simulink model "main"  (R2021a)
settings: Solver=ode113  StartTime=0.0  StopTime=100  RelTol=1e-13  AbsTol=1e-14
undefined symbols (not defined in the file or in its folder): Earth, initCond, Sensors, Spacecraft
libraries: aerolibutil x48, vrlib x31, dspsrcs4 x29, simulink x10, SADlibrary x8, commfilt2 x3, sharedtransform x3, dspfdesign x3, sharedutil x2, sharedTrackingLibrary x2, dspmathops x1
(part 2 of 3)

== system main/Subsystem1/Sun sensor reading3 ==
  True Sun position [body reference frame][km] : Inport  OutDataTypeStr=double  Unit=km
  q_S/B : Inport  Port=2
  Atan3 : Trigonometry  Operator=atan2
  Atan4 : Trigonometry  Operator=atan2
  Demux2 : Demux  Outputs=3
  Mux1 : Mux  Inputs=2
  Normalize Vector : vrlib/Utilities/Normalize Vector  maxzero=0
  Quaternion Rotation : aerolibutil/Quaternion Rotation
  Saturation1 : Saturate  UpperLimit=Sensors.sunSensor.fow  LowerLimit=-Sensors.sunSensor.fow
  Subsystem : Subsystem
  Zero-Order Hold : ZeroOrderHold  SampleTime=1/Sensors.sunSensor.freq
  Sun angles position [sensor axis] : Outport  OutDataTypeStr=double  Unit=1
  wires:
  True Sun position [body reference frame][km]/1 -> Zero-Order Hold/1
  q_S/B/1 -> Quaternion Rotation/1
  Zero-Order Hold/1 -> Normalize Vector/1
  Normalize Vector/1 -> Quaternion Rotation/2
  Quaternion Rotation/1 -> Subsystem/1(vec)
  Demux2/3 -> Atan3/2, Atan4/2
  Demux2/1 -> Atan4/1
  Atan4/1 -> Mux1/1
  Atan3/1 -> Mux1/2
  Mux1/1 -> Saturation1/1
  Subsystem/1(vec_rot) -> Demux2/1
  Demux2/2 -> Atan3/1
  Saturation1/1 -> Sun angles position [sensor axis]/1

== system main/Subsystem1/Sun sensor reading4 ==
  True Sun position [body reference frame][km] : Inport  OutDataTypeStr=double  Unit=km
  q_S/B : Inport  Port=2
  Atan3 : Trigonometry  Operator=atan2
  Atan4 : Trigonometry  Operator=atan2
  Demux2 : Demux  Outputs=3
  Mux1 : Mux  Inputs=2
  Normalize Vector : vrlib/Utilities/Normalize Vector  maxzero=0
  Quaternion Rotation : aerolibutil/Quaternion Rotation
  Saturation1 : Saturate  UpperLimit=Sensors.sunSensor.fow  LowerLimit=-Sensors.sunSensor.fow
  Subsystem : Subsystem
  Zero-Order Hold : ZeroOrderHold  SampleTime=1/Sensors.sunSensor.freq
  Sun angles position [sensor axis] : Outport  OutDataTypeStr=double  Unit=1
  wires:
  True Sun position [body reference frame][km]/1 -> Zero-Order Hold/1
  q_S/B/1 -> Quaternion Rotation/1
  Zero-Order Hold/1 -> Normalize Vector/1
  Normalize Vector/1 -> Quaternion Rotation/2
  Quaternion Rotation/1 -> Subsystem/1(vec)
  Demux2/3 -> Atan3/2, Atan4/2
  Demux2/1 -> Atan4/1
  Atan4/1 -> Mux1/1
  Atan3/1 -> Mux1/2
  Mux1/1 -> Saturation1/1
  Subsystem/1(vec_rot) -> Demux2/1
  Demux2/2 -> Atan3/1
  Saturation1/1 -> Sun angles position [sensor axis]/1

== system main/Subsystem1/Sun sensor reading5 ==
  True Sun position [body reference frame][km] : Inport  OutDataTypeStr=double  Unit=km
  q_S/B : Inport  Port=2
  Atan3 : Trigonometry  Operator=atan2
  Atan4 : Trigonometry  Operator=atan2
  Demux2 : Demux  Outputs=3
  Mux1 : Mux  Inputs=2
  Normalize Vector : vrlib/Utilities/Normalize Vector  maxzero=0
  Quaternion Rotation : aerolibutil/Quaternion Rotation
  Saturation1 : Saturate  UpperLimit=Sensors.sunSensor.fow  LowerLimit=-Sensors.sunSensor.fow
  Subsystem : Subsystem
  Zero-Order Hold : ZeroOrderHold  SampleTime=1/Sensors.sunSensor.freq
  Sun angles position [sensor axis] : Outport  OutDataTypeStr=double  Unit=1
  wires:
  True Sun position [body reference frame][km]/1 -> Zero-Order Hold/1
  q_S/B/1 -> Quaternion Rotation/1
  Zero-Order Hold/1 -> Normalize Vector/1
  Normalize Vector/1 -> Quaternion Rotation/2
  Quaternion Rotation/1 -> Subsystem/1(vec)
  Demux2/3 -> Atan3/2, Atan4/2
  Demux2/1 -> Atan4/1
  Atan4/1 -> Mux1/1
  Atan3/1 -> Mux1/2
  Mux1/1 -> Saturation1/1
  Subsystem/1(vec_rot) -> Demux2/1
  Demux2/2 -> Atan3/1
  Saturation1/1 -> Sun angles position [sensor axis]/1

== system main/Real physics/Air drag/Air density ==
  note: Because the density is a continuous function it doesn't matter if with an Height equal to a breakpoint value (e.g. =700km) we consider a base height of 700km or a base height of 600km
  Height : Inport
  1-D Lookup Base height : Lookup_n-D  NumberOfTableDimensions=1  BreakpointsForDimension1=Earth.atm_referenceHeight  IndexSearchMethod=Evenly spaced points  BeginIndexSearchUsingPreviousIndexResult=on  Table=Earth.atm_referenceHeight  InterpMethod=Flat  ExtrapMethod=Clip  UseLastTableValue=on  InternalRulePriority=Speed  RndMeth=Simplest  InputSameDT=on
  1-D Lookup Nominal density : Lookup_n-D  NumberOfTableDimensions=1  BreakpointsForDimension1=Earth.atm_referenceHeight  IndexSearchMethod=Evenly spaced points  BeginIndexSearchUsingPreviousIndexResult=on  Table=Earth.atm_nominalDensity  InterpMethod=Flat  InternalRulePriority=Speed  RndMeth=Simplest  InputSameDT=on
  1-D Lookup Scale height : Lookup_n-D  NumberOfTableDimensions=1  BreakpointsForDimension1=Earth.atm_referenceHeight  IndexSearchMethod=Evenly spaced points  BeginIndexSearchUsingPreviousIndexResult=on  Table=Earth.atm_scaleHeight  InterpMethod=Flat  InternalRulePriority=Speed  RndMeth=Simplest  InputSameDT=on
  Divide : Product  Inputs=*/
  Exp : Math  SaturateOnIntegerOverflow=on
  Product : Product
  Sum : Sum  Inputs=-+|
  Air density : Outport
  wires:
  Height/1 -> 1-D Lookup Nominal density/1, 1-D Lookup Scale height/1, 1-D Lookup Base height/1, Sum/1
  1-D Lookup Nominal density/1 -> Product/2
  1-D Lookup Base height/1 -> Sum/2
  Sum/1 -> Divide/1
  1-D Lookup Scale height/1 -> Divide/2
  Divide/1 -> Exp/1
  Product/1 -> Air density/1
  Exp/1 -> Product/1

== system main/Real physics/Magnetic dipole/Subsystem2 ==
  q_A/B : Inport
  r_NF : Inport  Port=2
  Clock : Clock
  Gain : Gain  Gain=2*pi/Earth.siderealDay
  MATLAB Function : MATLAB Function  TreatAsAtomicUnit=on
  MATLAB Function1 : MATLAB Function  TreatAsAtomicUnit=on
  Mux : Mux  Inputs=3
  Quaternion Conjugate : aerolibutil/Quaternion Conjugate
      settings: SourceProductBaseCode=AE
  Quaternion Rotation : aerolibutil/Quaternion Rotation
  Subsystem : Subsystem
  Subsystem1 : Subsystem
  B [BF] : Outport
  wires:
  q_A/B/1 -> Subsystem/1(q_A/B)
  Clock/1 -> Gain/1
  MATLAB Function/1(Bth) -> Mux/1
  Quaternion Conjugate/1 -> Subsystem/2(q_B/C)
  r_NF/1 -> MATLAB Function1/1(r_NF)
  Gain/1 -> MATLAB Function/1(RAGreenwich)
  MATLAB Function/2(Bph) -> Mux/2
  MATLAB Function1/1(RA) -> MATLAB Function/2(RA), Subsystem1/1(RA)
  Mux/1 -> Quaternion Rotation/2
  MATLAB Function1/2(dec) -> MATLAB Function/3(dec), Subsystem1/2(dec)
  MATLAB Function1/3(r) -> MATLAB Function/4(r)
  Subsystem1/1(q_T/N) -> Quaternion Conjugate/1
  Quaternion Rotation/1 -> B [BF]/1
  Subsystem/1(q_A/C) -> Quaternion Rotation/1  "Attitude error"
  MATLAB Function/3(Br) -> Mux/3

== system main/Real physics/Rotational dynamic/Euler equations (rigid body)  ==
  note: $\dot\mathbf{\Gamma} = \left[ (-I_z+I_y) \omega_y \omega_z \quad (-I_x+I_z) \omega_z \omega_x \quad \right (-I_y+I_x) \omega_x \omega_y]^T$
      |
      | Please note that
      | $\left[b \quad c \quad a \right] = \text{Cycle_3_vector}\left([a \quad b \quad c]\right)$
  omega [body reference frame] : Inport
  External torque [body reference frame] : Inport  Port=2  Unit=N*m
  Constant : Constant  Value=Spacecraft.str.inertia
  Cycle vector{,1..3} (4 alike) : SADlibrary/Cycle vector  SystemSampleTime=-1  VariantActivationTime=update diagram  Latency=0  AutoFrameSizeCalculation=off
  Divide : Product  Inputs=*/
  Product : Product  Inputs=3
  Sum : Sum  Inputs=++|
  Sum1 : Sum  Inputs=|-+
  omega dot [body reference frame] : Outport
  wires:
  Constant/1 -> Cycle vector2/1, Divide/2
  External torque [body reference frame]/1 -> Sum/1
  Sum/1 -> Divide/1
  Divide/1 -> omega dot [body reference frame]/1
  omega [body reference frame]/1 -> Cycle vector/1
  Cycle vector2/1 -> Cycle vector3/1, Sum1/1
  Cycle vector3/1 -> Sum1/2
  Cycle vector/1 -> Cycle vector1/1, Product/2
  Cycle vector1/1 -> Product/1
  Sum1/1 -> Product/3
  Product/1 -> Sum/2

== system main/Real physics/Rotational dynamic/Kinematics with quaternions ==
  q_I/N : Inport  Unit=1
  omega [IF] : Inport  Port=2  Unit=rad/s
  Gain1 : Gain  Gain=1/2
  MATLAB Function1 : MATLAB Function  TreatAsAtomicUnit=on
  Matrix Multiply : Product  Multiplication=Matrix(*)
  q_I/N_dot : Outport
  wires:
  omega [IF]/1 -> MATLAB Function1/1(omega)
  Gain1/1 -> Matrix Multiply/1
  Matrix Multiply/1 -> q_I/N_dot/1
  MATLAB Function1/1(Omega) -> Gain1/1
  q_I/N/1 -> Matrix Multiply/2

== system main/Real physics/Rotational dynamic/getGamma0 ==
  Constant1 : Constant  Value=Spacecraft.initialKepElm.a  VectorParams1D=off
  Constant3 : Constant  Value=Spacecraft.initialKepElm.e
  Constant4 : Constant  Value=Spacecraft.initialKepElm.i
  Constant5 : Constant  Value=Spacecraft.initialKepElm.Omega
  Constant6 : Constant  Value=Spacecraft.initialKepElm.f
  Constant8 : Constant  Value=Spacecraft.initialKepElm.omega
  MATLAB Function3 : MATLAB Function  TreatAsAtomicUnit=on
  MATLAB Function4 : MATLAB Function  TreatAsAtomicUnit=on
  Terminator : Terminator
  Gamma0 : Outport
  wires:
  Constant5/1 -> MATLAB Function3/4(Omega)
  MATLAB Function4/1(Gamma0) -> Gamma0/1
  Constant6/1 -> MATLAB Function3/6(f)
  Constant8/1 -> MATLAB Function3/5(omega)
  MATLAB Function3/1(r) -> Terminator/1
  Constant1/1 -> MATLAB Function3/1(a)
  MATLAB Function3/2(v) -> MATLAB Function4/1(vG0)
  Constant4/1 -> MATLAB Function3/3(i)
  Constant3/1 -> MATLAB Function3/2(e)

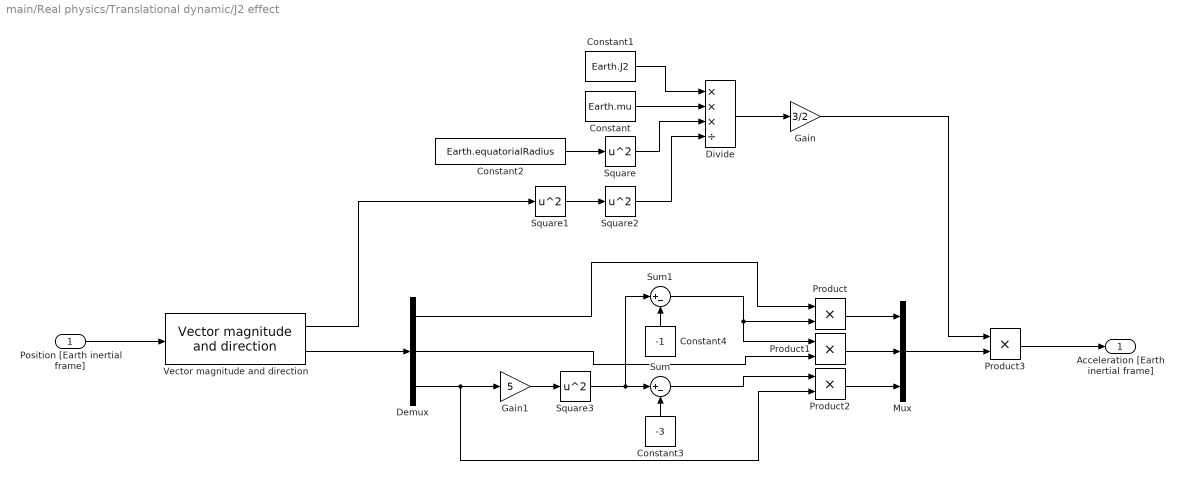
== system main/Real physics/Translational dynamic/J2 effect ==
  Position [Earth inertial frame] : Inport
  Constant : Constant  Value=Earth.mu
  Constant1 : Constant  Value=Earth.J2
  Constant2 : Constant  Value=Earth.equatorialRadius
  Constant3 : Constant  Value=-3
  Constant4 : Constant  Value=-1
  Demux : Demux  Outputs=3
  Divide : Product  Inputs=***/
  Gain : Gain  Gain=3/2
  Gain1 : Gain  Gain=5
  Mux : Mux  Inputs=3
  Product{,1..3} (4 alike) : Product
  Square{,1..3} (4 alike) : Math  Operator=square  SaturateOnIntegerOverflow=on
  Sum : Sum  Inputs=|+-
  Sum1 : Sum  Inputs=|+-
  Vector magnitude and direction : SADlibrary/Vector magnitude and direction  SystemSampleTime=-1  VariantActivationTime=update diagram  Latency=0  AutoFrameSizeCalculation=off
  Acceleration [Earth inertial frame] : Outport
  wires:
  Constant2/1 -> Square/1
  Constant1/1 -> Divide/1
  Constant/1 -> Divide/2
  Square/1 -> Divide/3
  Divide/1 -> Gain/1
  Square1/1 -> Square2/1
  Square2/1 -> Divide/4
  Vector magnitude and direction/1 -> Square1/1
  Position [Earth inertial frame]/1 -> Vector magnitude and direction/1
  Vector magnitude and direction/2 -> Demux/1
  Demux/3 -> Product2/2, Gain1/1
  Gain1/1 -> Square3/1
  Square3/1 -> Sum1/1, Sum/1
  Constant3/1 -> Sum/2
  Constant4/1 -> Sum1/2
  Product/1 -> Mux/1
  Product1/1 -> Mux/2
  Product2/1 -> Mux/3
  Sum1/1 -> Product1/1, Product/2
  Demux/1 -> Product/1
  Demux/2 -> Product1/2
  Sum/1 -> Product2/1
  Mux/1 -> Product3/2
  Product3/1 -> Acceleration [Earth inertial frame]/1
  Gain/1 -> Product3/1

== system main/Real physics/Translational dynamic/Main contribution ==
  Position [Earth inertial frame] : Inport
  Constant : Constant  Value=Earth.mu
  Divide : Product  Inputs=*/
  Gain : Gain  Gain=-1
  Product : Product
  Square : Math  Operator=square  SaturateOnIntegerOverflow=on
  Vector magnitude and direction : SADlibrary/Vector magnitude and direction  SystemSampleTime=-1  VariantActivationTime=update diagram  Latency=0  AutoFrameSizeCalculation=off
  Acceleration [Earth inertial frame] : Outport
  wires:
  Square/1 -> Divide/2
  Product/1 -> Acceleration [Earth inertial frame]/1
  Position [Earth inertial frame]/1 -> Vector magnitude and direction/1
  Divide/1 -> Gain/1
  Constant/1 -> Divide/1
  Vector magnitude and direction/1 -> Square/1
  Vector magnitude and direction/2 -> Product/2
  Gain/1 -> Product/1

== system main/Star sensor/Vector 2 angles/Subsystem ==
  vec : Inport
  Constant : Constant  Value=[0 0 1]
  Cross Product : vrlib/Utilities/Cross Product
  MATLAB Function : MATLAB Function  TreatAsAtomicUnit=on
  MATLAB Function1 : MATLAB Function  TreatAsAtomicUnit=on
  Normalize Vector1 : vrlib/Utilities/Normalize Vector  maxzero=0
  Quaternion Rotation : aerolibutil/Quaternion Rotation
  Quaternion Rotation1 : aerolibutil/Quaternion Rotation
  Random Source1 : dspsrcs4/Random Source  SrcType=Gaussian  NormMethod=Ziggurat  CltLength=12  MinVal=0  MaxVal=1  MeanVal=0  VarVal=Sensors.starTracker.aboutBoresight  RepMode=Not repeatable  rawSeed=1  IsInherit=off  SampMode=Discrete  SampTime=1/Sensors.starTracker.freq  SampFrame=1  DataType=Double  OutComplex=Real  OutputFrames=off
  Random Source2 : dspsrcs4/Random Source  SrcType=Gaussian  NormMethod=Ziggurat  CltLength=12  MinVal=0  MaxVal=1  MeanVal=0  VarVal=Sensors.starTracker.crossBoresight  RepMode=Not repeatable  rawSeed=1  IsInherit=off  SampMode=Discrete  SampTime=1/Sensors.starTracker.freq  SampFrame=1  DataType=Double  OutComplex=Real  OutputFrames=off
  vec_rot : Outport
  wires:
  vec/1 -> Quaternion Rotation/2
  Quaternion Rotation1/1 -> vec_rot/1
  MATLAB Function1/1(q) -> Quaternion Rotation1/1
  Random Source2/1 -> MATLAB Function1/1(theta)
  Quaternion Rotation/1 -> Cross Product/2, Quaternion Rotation1/2
  MATLAB Function/1(q) -> Quaternion Rotation/1
  Random Source1/1 -> MATLAB Function/1(theta)
  Constant/1 -> Cross Product/1
  Cross Product/1 -> Normalize Vector1/1
  Normalize Vector1/1 -> MATLAB Function1/2(e)

== system main/Star sensor/Vector 2 angles1/Subsystem ==
  vec : Inport
  Constant : Constant  Value=[0 0 1]
  Cross Product : vrlib/Utilities/Cross Product
  MATLAB Function : MATLAB Function  TreatAsAtomicUnit=on
  MATLAB Function1 : MATLAB Function  TreatAsAtomicUnit=on
  Normalize Vector : vrlib/Utilities/Normalize Vector  Commented=on  maxzero=0
  Normalize Vector1 : vrlib/Utilities/Normalize Vector  maxzero=0
  Quaternion Rotation : aerolibutil/Quaternion Rotation
  Quaternion Rotation1 : aerolibutil/Quaternion Rotation
  Random Source1 : dspsrcs4/Random Source  SrcType=Gaussian  NormMethod=Ziggurat  CltLength=12  MinVal=0  MaxVal=1  MeanVal=0  VarVal=Sensors.starTracker.aboutBoresight  RepMode=Not repeatable  rawSeed=1  IsInherit=off  SampMode=Discrete  SampTime=1/Sensors.starTracker.freq  SampFrame=1  DataType=Double  OutComplex=Real  OutputFrames=off
  Random Source2 : dspsrcs4/Random Source  SrcType=Gaussian  NormMethod=Ziggurat  CltLength=12  MinVal=0  MaxVal=1  MeanVal=0  VarVal=Sensors.starTracker.crossBoresight  RepMode=Not repeatable  rawSeed=1  IsInherit=off  SampMode=Discrete  SampTime=1/Sensors.starTracker.freq  SampFrame=1  DataType=Double  OutComplex=Real  OutputFrames=off
  Random Source3 : dspsrcs4/Random Source  Commented=on  SrcType=Uniform  NormMethod=Ziggurat  CltLength=12  MinVal=0  MaxVal=1  MeanVal=0  VarVal=1  RepMode=Not repeatable  rawSeed=1  IsInherit=off  SampMode=Discrete  SampTime=1/Sensors.starTracker.freq  SampFrame=2  DataType=Double  OutComplex=Real  OutputFrames=off
  vec_rot : Outport
  wires:
  vec/1 -> Quaternion Rotation/2
  Random Source3/1 -> Normalize Vector/1
  Normalize Vector/1 -> ?
  Quaternion Rotation1/1 -> vec_rot/1
  MATLAB Function1/1(q) -> Quaternion Rotation1/1
  Random Source2/1 -> MATLAB Function1/1(theta)
  Quaternion Rotation/1 -> Cross Product/2, Quaternion Rotation1/2
  MATLAB Function/1(q) -> Quaternion Rotation/1
  Random Source1/1 -> MATLAB Function/1(theta)
  Constant/1 -> Cross Product/1
  Cross Product/1 -> Normalize Vector1/1
  Normalize Vector1/1 -> MATLAB Function1/2(e)

== system main/Star sensor/Vector 2 angles2/Subsystem ==
  vec : Inport
  Constant : Constant  Value=[0 0 1]
  Cross Product : vrlib/Utilities/Cross Product
  MATLAB Function : MATLAB Function  TreatAsAtomicUnit=on
  MATLAB Function1 : MATLAB Function  TreatAsAtomicUnit=on
  Normalize Vector : vrlib/Utilities/Normalize Vector  Commented=on  maxzero=0
  Normalize Vector1 : vrlib/Utilities/Normalize Vector  maxzero=0
  Quaternion Rotation : aerolibutil/Quaternion Rotation
  Quaternion Rotation1 : aerolibutil/Quaternion Rotation
  Random Source1 : dspsrcs4/Random Source  SrcType=Gaussian  NormMethod=Ziggurat  CltLength=12  MinVal=0  MaxVal=1  MeanVal=0  VarVal=Sensors.starTracker.aboutBoresight  RepMode=Not repeatable  rawSeed=1  IsInherit=off  SampMode=Discrete  SampTime=1/Sensors.starTracker.freq  SampFrame=1  DataType=Double  OutComplex=Real  OutputFrames=off
  Random Source2 : dspsrcs4/Random Source  SrcType=Gaussian  NormMethod=Ziggurat  CltLength=12  MinVal=0  MaxVal=1  MeanVal=0  VarVal=Sensors.starTracker.crossBoresight  RepMode=Not repeatable  rawSeed=1  IsInherit=off  SampMode=Discrete  SampTime=1/Sensors.starTracker.freq  SampFrame=1  DataType=Double  OutComplex=Real  OutputFrames=off
  Random Source3 : dspsrcs4/Random Source  Commented=on  SrcType=Uniform  NormMethod=Ziggurat  CltLength=12  MinVal=0  MaxVal=1  MeanVal=0  VarVal=1  RepMode=Not repeatable  rawSeed=1  IsInherit=off  SampMode=Discrete  SampTime=1/Sensors.starTracker.freq  SampFrame=2  DataType=Double  OutComplex=Real  OutputFrames=off
  vec_rot : Outport
  wires:
  vec/1 -> Quaternion Rotation/2
  Random Source3/1 -> Normalize Vector/1
  Normalize Vector/1 -> ?
  Quaternion Rotation1/1 -> vec_rot/1
  MATLAB Function1/1(q) -> Quaternion Rotation1/1
  Random Source2/1 -> MATLAB Function1/1(theta)
  Quaternion Rotation/1 -> Cross Product/2, Quaternion Rotation1/2
  MATLAB Function/1(q) -> Quaternion Rotation/1
  Random Source1/1 -> MATLAB Function/1(theta)
  Constant/1 -> Cross Product/1
  Cross Product/1 -> Normalize Vector1/1
  Normalize Vector1/1 -> MATLAB Function1/2(e)

== system main/Star sensor/Vector 2 angles3/Subsystem ==
  vec : Inport
  Constant : Constant  Value=[0 0 1]
  Cross Product : vrlib/Utilities/Cross Product
  MATLAB Function : MATLAB Function  TreatAsAtomicUnit=on
  MATLAB Function1 : MATLAB Function  TreatAsAtomicUnit=on
  Normalize Vector : vrlib/Utilities/Normalize Vector  Commented=on  maxzero=0
  Normalize Vector1 : vrlib/Utilities/Normalize Vector  maxzero=0
  Quaternion Rotation : aerolibutil/Quaternion Rotation
  Quaternion Rotation1 : aerolibutil/Quaternion Rotation
  Random Source1 : dspsrcs4/Random Source  SrcType=Gaussian  NormMethod=Ziggurat  CltLength=12  MinVal=0  MaxVal=1  MeanVal=0  VarVal=Sensors.starTracker.aboutBoresight  RepMode=Not repeatable  rawSeed=1  IsInherit=off  SampMode=Discrete  SampTime=1/Sensors.starTracker.freq  SampFrame=1  DataType=Double  OutComplex=Real  OutputFrames=off
  Random Source2 : dspsrcs4/Random Source  SrcType=Gaussian  NormMethod=Ziggurat  CltLength=12  MinVal=0  MaxVal=1  MeanVal=0  VarVal=Sensors.starTracker.crossBoresight  RepMode=Not repeatable  rawSeed=1  IsInherit=off  SampMode=Discrete  SampTime=1/Sensors.starTracker.freq  SampFrame=1  DataType=Double  OutComplex=Real  OutputFrames=off
  Random Source3 : dspsrcs4/Random Source  Commented=on  SrcType=Uniform  NormMethod=Ziggurat  CltLength=12  MinVal=0  MaxVal=1  MeanVal=0  VarVal=1  RepMode=Not repeatable  rawSeed=1  IsInherit=off  SampMode=Discrete  SampTime=1/Sensors.starTracker.freq  SampFrame=2  DataType=Double  OutComplex=Real  OutputFrames=off
  vec_rot : Outport
  wires:
  vec/1 -> Quaternion Rotation/2
  Random Source3/1 -> Normalize Vector/1
  Normalize Vector/1 -> ?
  Quaternion Rotation1/1 -> vec_rot/1
  MATLAB Function1/1(q) -> Quaternion Rotation1/1
  Random Source2/1 -> MATLAB Function1/1(theta)
  Quaternion Rotation/1 -> Cross Product/2, Quaternion Rotation1/2
  MATLAB Function/1(q) -> Quaternion Rotation/1
  Random Source1/1 -> MATLAB Function/1(theta)
  Constant/1 -> Cross Product/1
  Cross Product/1 -> Normalize Vector1/1
  Normalize Vector1/1 -> MATLAB Function1/2(e)

== system main/Subsystem1/Sun sensor reading/Subsystem ==
  vec : Inport
  Constant : Constant  Value=[0 0 1]
  Cross Product : vrlib/Utilities/Cross Product
  MATLAB Function : MATLAB Function  TreatAsAtomicUnit=on
  MATLAB Function2 : MATLAB Function  TreatAsAtomicUnit=on
  Normalize Vector1 : vrlib/Utilities/Normalize Vector  maxzero=0
  Quaternion Rotation : aerolibutil/Quaternion Rotation
  Quaternion Rotation1 : aerolibutil/Quaternion Rotation
  Random Source1 : dspsrcs4/Random Source  SrcType=Gaussian  NormMethod=Ziggurat  CltLength=12  MinVal=0  MaxVal=1  MeanVal=0  VarVal=Sensors.sunSensor.aboutBoresight  RepMode=Not repeatable  rawSeed=1  IsInherit=off  SampMode=Discrete  SampTime=1/Sensors.sunSensor.freq  SampFrame=1  DataType=Double  OutComplex=Real  OutputFrames=off
  Random Source2 : dspsrcs4/Random Source  SrcType=Gaussian  NormMethod=Ziggurat  CltLength=12  MinVal=0  MaxVal=1  MeanVal=0  VarVal=Sensors.sunSensor.crossBoresight  RepMode=Not repeatable  rawSeed=1  IsInherit=off  SampMode=Discrete  SampTime=1/Sensors.sunSensor.freq  SampFrame=1  DataType=Double  OutComplex=Real  OutputFrames=off
  vec_rot : Outport
  wires:
  vec/1 -> Quaternion Rotation/2
  Quaternion Rotation1/1 -> vec_rot/1
  MATLAB Function/1(q) -> Quaternion Rotation/1
  Random Source1/1 -> MATLAB Function/1(theta)
  Normalize Vector1/1 -> MATLAB Function2/2(e)
  Quaternion Rotation/1 -> Quaternion Rotation1/2, Cross Product/2
  Random Source2/1 -> MATLAB Function2/1(theta)
  MATLAB Function2/1(q) -> Quaternion Rotation1/1
  Constant/1 -> Cross Product/1
  Cross Product/1 -> Normalize Vector1/1

== system main/Subsystem1/Sun sensor reading1/Subsystem ==
  vec : Inport
  Constant : Constant  Value=[0 0 1]
  Cross Product : vrlib/Utilities/Cross Product
  MATLAB Function : MATLAB Function  TreatAsAtomicUnit=on
  MATLAB Function2 : MATLAB Function  TreatAsAtomicUnit=on
  Normalize Vector1 : vrlib/Utilities/Normalize Vector  maxzero=0
  Quaternion Rotation : aerolibutil/Quaternion Rotation
  Quaternion Rotation1 : aerolibutil/Quaternion Rotation
  Random Source1 : dspsrcs4/Random Source  SrcType=Gaussian  NormMethod=Ziggurat  CltLength=12  MinVal=0  MaxVal=1  MeanVal=0  VarVal=Sensors.sunSensor.aboutBoresight  RepMode=Not repeatable  rawSeed=1  IsInherit=off  SampMode=Discrete  SampTime=1/Sensors.sunSensor.freq  SampFrame=1  DataType=Double  OutComplex=Real  OutputFrames=off
  Random Source2 : dspsrcs4/Random Source  SrcType=Gaussian  NormMethod=Ziggurat  CltLength=12  MinVal=0  MaxVal=1  MeanVal=0  VarVal=Sensors.sunSensor.crossBoresight  RepMode=Not repeatable  rawSeed=1  IsInherit=off  SampMode=Discrete  SampTime=1/Sensors.sunSensor.freq  SampFrame=1  DataType=Double  OutComplex=Real  OutputFrames=off
  vec_rot : Outport
  wires:
  vec/1 -> Quaternion Rotation/2
  Quaternion Rotation1/1 -> vec_rot/1
  MATLAB Function/1(q) -> Quaternion Rotation/1
  Random Source1/1 -> MATLAB Function/1(theta)
  Normalize Vector1/1 -> MATLAB Function2/2(e)
  Quaternion Rotation/1 -> Quaternion Rotation1/2, Cross Product/2
  Random Source2/1 -> MATLAB Function2/1(theta)
  MATLAB Function2/1(q) -> Quaternion Rotation1/1
  Constant/1 -> Cross Product/1
  Cross Product/1 -> Normalize Vector1/1

== system main/Subsystem1/Sun sensor reading2/Subsystem ==
  vec : Inport
  Constant : Constant  Value=[0 0 1]
  Cross Product : vrlib/Utilities/Cross Product
  MATLAB Function : MATLAB Function  TreatAsAtomicUnit=on
  MATLAB Function2 : MATLAB Function  TreatAsAtomicUnit=on
  Normalize Vector1 : vrlib/Utilities/Normalize Vector  maxzero=0
  Quaternion Rotation : aerolibutil/Quaternion Rotation
  Quaternion Rotation1 : aerolibutil/Quaternion Rotation
  Random Source1 : dspsrcs4/Random Source  SrcType=Gaussian  NormMethod=Ziggurat  CltLength=12  MinVal=0  MaxVal=1  MeanVal=0  VarVal=Sensors.sunSensor.aboutBoresight  RepMode=Not repeatable  rawSeed=1  IsInherit=off  SampMode=Discrete  SampTime=1/Sensors.sunSensor.freq  SampFrame=1  DataType=Double  OutComplex=Real  OutputFrames=off
  Random Source2 : dspsrcs4/Random Source  SrcType=Gaussian  NormMethod=Ziggurat  CltLength=12  MinVal=0  MaxVal=1  MeanVal=0  VarVal=Sensors.sunSensor.crossBoresight  RepMode=Not repeatable  rawSeed=1  IsInherit=off  SampMode=Discrete  SampTime=1/Sensors.sunSensor.freq  SampFrame=1  DataType=Double  OutComplex=Real  OutputFrames=off
  vec_rot : Outport
  wires:
  vec/1 -> Quaternion Rotation/2
  Quaternion Rotation1/1 -> vec_rot/1
  MATLAB Function/1(q) -> Quaternion Rotation/1
  Random Source1/1 -> MATLAB Function/1(theta)
  Normalize Vector1/1 -> MATLAB Function2/2(e)
  Quaternion Rotation/1 -> Quaternion Rotation1/2, Cross Product/2
  Random Source2/1 -> MATLAB Function2/1(theta)
  MATLAB Function2/1(q) -> Quaternion Rotation1/1
  Constant/1 -> Cross Product/1
  Cross Product/1 -> Normalize Vector1/1

== system main/Subsystem1/Sun sensor reading3/Subsystem ==
  vec : Inport
  Constant : Constant  Value=[0 0 1]
  Cross Product : vrlib/Utilities/Cross Product
  MATLAB Function : MATLAB Function  TreatAsAtomicUnit=on
  MATLAB Function2 : MATLAB Function  TreatAsAtomicUnit=on
  Normalize Vector1 : vrlib/Utilities/Normalize Vector  maxzero=0
  Quaternion Rotation : aerolibutil/Quaternion Rotation
  Quaternion Rotation1 : aerolibutil/Quaternion Rotation
  Random Source1 : dspsrcs4/Random Source  SrcType=Gaussian  NormMethod=Ziggurat  CltLength=12  MinVal=0  MaxVal=1  MeanVal=0  VarVal=Sensors.sunSensor.aboutBoresight  RepMode=Not repeatable  rawSeed=1  IsInherit=off  SampMode=Discrete  SampTime=1/Sensors.sunSensor.freq  SampFrame=1  DataType=Double  OutComplex=Real  OutputFrames=off
  Random Source2 : dspsrcs4/Random Source  SrcType=Gaussian  NormMethod=Ziggurat  CltLength=12  MinVal=0  MaxVal=1  MeanVal=0  VarVal=Sensors.sunSensor.crossBoresight  RepMode=Not repeatable  rawSeed=1  IsInherit=off  SampMode=Discrete  SampTime=1/Sensors.sunSensor.freq  SampFrame=1  DataType=Double  OutComplex=Real  OutputFrames=off
  vec_rot : Outport
  wires:
  vec/1 -> Quaternion Rotation/2
  Quaternion Rotation1/1 -> vec_rot/1
  MATLAB Function/1(q) -> Quaternion Rotation/1
  Random Source1/1 -> MATLAB Function/1(theta)
  Normalize Vector1/1 -> MATLAB Function2/2(e)
  Quaternion Rotation/1 -> Quaternion Rotation1/2, Cross Product/2
  Random Source2/1 -> MATLAB Function2/1(theta)
  MATLAB Function2/1(q) -> Quaternion Rotation1/1
  Constant/1 -> Cross Product/1
  Cross Product/1 -> Normalize Vector1/1

== system main/Subsystem1/Sun sensor reading4/Subsystem ==
  vec : Inport
  Constant : Constant  Value=[0 0 1]
  Cross Product : vrlib/Utilities/Cross Product
  MATLAB Function : MATLAB Function  TreatAsAtomicUnit=on
  MATLAB Function2 : MATLAB Function  TreatAsAtomicUnit=on
  Normalize Vector1 : vrlib/Utilities/Normalize Vector  maxzero=0
  Quaternion Rotation : aerolibutil/Quaternion Rotation
  Quaternion Rotation1 : aerolibutil/Quaternion Rotation
  Random Source1 : dspsrcs4/Random Source  SrcType=Gaussian  NormMethod=Ziggurat  CltLength=12  MinVal=0  MaxVal=1  MeanVal=0  VarVal=Sensors.sunSensor.aboutBoresight  RepMode=Not repeatable  rawSeed=1  IsInherit=off  SampMode=Discrete  SampTime=1/Sensors.sunSensor.freq  SampFrame=1  DataType=Double  OutComplex=Real  OutputFrames=off
  Random Source2 : dspsrcs4/Random Source  SrcType=Gaussian  NormMethod=Ziggurat  CltLength=12  MinVal=0  MaxVal=1  MeanVal=0  VarVal=Sensors.sunSensor.crossBoresight  RepMode=Not repeatable  rawSeed=1  IsInherit=off  SampMode=Discrete  SampTime=1/Sensors.sunSensor.freq  SampFrame=1  DataType=Double  OutComplex=Real  OutputFrames=off
  vec_rot : Outport
  wires:
  vec/1 -> Quaternion Rotation/2
  Quaternion Rotation1/1 -> vec_rot/1
  MATLAB Function/1(q) -> Quaternion Rotation/1
  Random Source1/1 -> MATLAB Function/1(theta)
  Normalize Vector1/1 -> MATLAB Function2/2(e)
  Quaternion Rotation/1 -> Quaternion Rotation1/2, Cross Product/2
  Random Source2/1 -> MATLAB Function2/1(theta)
  MATLAB Function2/1(q) -> Quaternion Rotation1/1
  Constant/1 -> Cross Product/1
  Cross Product/1 -> Normalize Vector1/1

== system main/Subsystem1/Sun sensor reading5/Subsystem ==
  vec : Inport
  Constant : Constant  Value=[0 0 1]
  Cross Product : vrlib/Utilities/Cross Product
  MATLAB Function : MATLAB Function  TreatAsAtomicUnit=on
  MATLAB Function2 : MATLAB Function  TreatAsAtomicUnit=on
  Normalize Vector1 : vrlib/Utilities/Normalize Vector  maxzero=0
  Quaternion Rotation : aerolibutil/Quaternion Rotation
  Quaternion Rotation1 : aerolibutil/Quaternion Rotation
  Random Source1 : dspsrcs4/Random Source  SrcType=Gaussian  NormMethod=Ziggurat  CltLength=12  MinVal=0  MaxVal=1  MeanVal=0  VarVal=Sensors.sunSensor.aboutBoresight  RepMode=Not repeatable  rawSeed=1  IsInherit=off  SampMode=Discrete  SampTime=1/Sensors.sunSensor.freq  SampFrame=1  DataType=Double  OutComplex=Real  OutputFrames=off
  Random Source2 : dspsrcs4/Random Source  SrcType=Gaussian  NormMethod=Ziggurat  CltLength=12  MinVal=0  MaxVal=1  MeanVal=0  VarVal=Sensors.sunSensor.crossBoresight  RepMode=Not repeatable  rawSeed=1  IsInherit=off  SampMode=Discrete  SampTime=1/Sensors.sunSensor.freq  SampFrame=1  DataType=Double  OutComplex=Real  OutputFrames=off
  vec_rot : Outport
  wires:
  vec/1 -> Quaternion Rotation/2
  Quaternion Rotation1/1 -> vec_rot/1
  MATLAB Function/1(q) -> Quaternion Rotation/1
  Random Source1/1 -> MATLAB Function/1(theta)
  Normalize Vector1/1 -> MATLAB Function2/2(e)
  Quaternion Rotation/1 -> Quaternion Rotation1/2, Cross Product/2
  Random Source2/1 -> MATLAB Function2/1(theta)
  MATLAB Function2/1(q) -> Quaternion Rotation1/1
  Constant/1 -> Cross Product/1
  Cross Product/1 -> Normalize Vector1/1

== system main/Real physics/Magnetic dipole/Subsystem2/Subsystem ==
  q_A/B : Inport
  q_B/C : Inport  Port=2
  Quaternion Multiplication : aerolibutil/Quaternion Multiplication
  q_A/C : Outport
  wires:
  q_A/B/1 -> Quaternion Multiplication/2
  q_B/C/1 -> Quaternion Multiplication/1
  Quaternion Multiplication/1 -> q_A/C/1

== system main/Real physics/Magnetic dipole/Subsystem2/Subsystem1 ==
  RA : Inport
  dec : Inport  Port=2
  MATLAB Function2 : MATLAB Function  TreatAsAtomicUnit=on
  MATLAB Function3 : MATLAB Function  TreatAsAtomicUnit=on
  Quaternion Multiplication : aerolibutil/Quaternion Multiplication
  q_T/N : Outport
  wires:
  Quaternion Multiplication/1 -> q_T/N/1
  RA/1 -> MATLAB Function2/1(RA)
  MATLAB Function3/1(q) -> Quaternion Multiplication/1
  dec/1 -> MATLAB Function3/1(dec)
  MATLAB Function2/1(q) -> Quaternion Multiplication/2

== matlab function main/Ideal control law/MATLAB Function ==
  data: J input; omegaBody input; omegaErr input; u output; qErr input
function u = lyapunovControl(J,omegaBody,omegaErr,qErr)
k1 = 1.73;
k2 = 0.5 * 1;

% 2.5e-3
u = -k1 * omegaErr -2*k2 * qErr(1)*qErr(2:4) + cross(omegaBody-omegaErr,J.*omegaBody);

== matlab function main/Ideal control law/MATLAB Function1 ==
  data: q input; e output
function e = fcn(q)

e = sqrt(q(2)^2+q(3)^2+q(4)^2) * 180 / pi * 2;

== matlab function main/MATLAB Function4 ==
  data: J input; omegaBody input; u output
function u = lyapunovDetumbling(J,omegaBody)
k1 = 100;

% 2.5e-3
% omegaB * JB * domegaB = omegaB * (JB * omegaB x omegaB + u)
u = -k1 * omegaBody + cross(omegaBody,J.*omegaBody);

== matlab function main/Solve Whabba's problem/MATLAB Function1 ==
  settings: updateMethod=DISCRETE
  data: K input; q output; qGuess input; err output
function [q,err] = getQ(K,qGuess)

q = qGuess;
err = 1;

for i=1:10 % err > 1e-6
    qOld = q;
    q = K*q;
    q = q/norm(q);
    err = sum((q - qOld).^2);
end

== matlab function main/Solve Whabba's problem/MATLAB Function2 ==
  data: S input; B output; V input
function B = computeBmatrix(S,V)%s1,v1,s2,v2,s3,v3)

B = zeros(3);%size(S,1));
for i=1:size(S,2)
    B = B + S(:,i)*V(:,i)';
end

% B = s1*v1'+s2*v2'+s3*v3';

== matlab function main/Solve Whabba's problem/MATLAB Function3 ==
  data: B input; A output
function A = BtoA(B)
[U,~,V] = svd(B);
M = diag([1 1 det(U)*det(V)]);
A = U*M*V';
%A = B \ sqrtm(B'*B);

== matlab function main/Ideal control law/MATLAB Function3 ==
  data: om input; e output
function e = fcn(om)

e = sqrt(om(1)^2+om(2)^2+om(3)^2) * 180 / pi * 2;

== matlab function main/Subsystem1/Sun sensor reading1/Subsystem/MATLAB Function ==
  data: theta input; q output
function q = aboutBoresightRotation(theta)

q = [cos(theta/2) 0 0 sin(theta/2)];

== matlab function main/Control allocator/MATLAB Function3 ==
  data: dt input; cgtTorque input size=[3 4]; dGammaId input size=3; xOpt output size=4
function xOpt = controlAllocator(dt,cgtTorque,dGammaId)

nThrusters = 4;
opt = optimoptions('lsqlin','Algorithm','active-set');
xOpt = lsqlin(cgtTorque,dGammaId,[],[],[],[],zeros(nThrusters,1),dt*ones(nThrusters,1),zeros(nThrusters,1),opt);

== matlab function main/Real physics/Translational dynamic/MATLAB Function ==
  data: a input; e input; f input; fDot output; mu input
function fDot = get_fDot(a,e,f,mu)

fDot = sqrt(mu)/(a*(1-e^2))^(3/2) * (1 + e*cos(f))^2;

== matlab function main/Real physics/Translational dynamic/MATLAB Function1 ==
  data: mu input; a input; r output; v output; e input; i input; Omega input; omega input; f input
function [r,v] = kep2car(mu,a,e,i,Omega,omega,f)
% Radial, transversal, out of plane versors (RSW frame) (See the appendix)
lat = asin( sin(f+omega).*sin(i) );
alpha = atan2( cos(i).*sin(f+omega), cos(f+omega) );
alpha = alpha + Omega;

R = [ cos(lat).*cos(alpha) ; ...
      cos(lat).*sin(alpha) ; ...
      sin(lat)             ];

W = [ sin(i).*sin(Omega)    ; ...
      sin(i).*(-cos(Omega)) ; ...
      cos(i)                ];

S = cross(W,R);

% Position vector
r = a.*(1-e.^2)./(1+e.*cos(f)) .* R;

% Velocity vector
v = sqrt(mu./(a.*(1-e.^2))) .* ( e.*sin(f).*R + ( 1+e.*cos(f) ).*S );

end

== matlab function main/Real physics/Rotational dynamic/MATLAB Function ==
  data: torque input; vG input; omega input; gammaDot output
function gammaDot = rotationalDynamics(torque,vG,omega)
m = Spacecraft.str.mass;
G_O = Spacecraft.str.com;

% vO = vG - ω x (G-O)
vO = vG - cross(omega,G_O);
gammaDot = torque - m*cross(vO,vG);

== stateflow chart main/Chart ==
  state State propagation
  state State1 correction
  (default) -> State propagation
  State propagation -> State1 correction
  State1 correction -> State propagation

== matlab function main/Real physics/Rotational dynamic/MATLAB Function1 ==
  data: J input; omega_IF input; omegaDot_IF output; torque_IF input
function omegaDot_IF = EulerEqn(J,omega_IF,torque_IF)

omegaDot_IF = zeros(3,1);

omegaDot_IF(1) = ((J(2)-J(3))*omega_IF(2)*omega_IF(3) + torque_IF(1))/J(1);
omegaDot_IF(2) = ((J(3)-J(1))*omega_IF(1)*omega_IF(3) + torque_IF(2))/J(2);
omegaDot_IF(3) = ((J(1)-J(2))*omega_IF(1)*omega_IF(2) + torque_IF(3))/J(3);

== matlab function main/Real physics/Rotational dynamic/MATLAB Function2 ==
  data: Gamma input; omega output; vG input
function omega = fromGammaToOmega(Gamma,vG)
m = Spacecraft.str.mass;
J = Spacecraft.str.inertia;
G_O = Spacecraft.str.com;

omega = J \ (Gamma - m*cross(G_O,vG));

== matlab function main/Real physics/Rotational dynamic/getGamma0/MATLAB Function3 ==
  data: a input; r output; v output; e input; i input; Omega input; omega input; f input
function [r,v] = kep2car(a,e,i,Omega,omega,f)
% Useful aliases
mu = Earth.mu;

% Actual code
% Radial, transversal, out of plane versors (RSW frame) (See the appendix)
lat = asin( sin(f+omega).*sin(i) );
alpha = atan2( cos(i).*sin(f+omega), cos(f+omega) );
alpha = alpha + Omega;

R = [ cos(lat).*cos(alpha) ; ...
      cos(lat).*sin(alpha) ; ...
      sin(lat)             ];

W = [ sin(i).*sin(Omega)    ; ...
      sin(i).*(-cos(Omega)) ; ...
      cos(i)                ];

S = cross(W,R);

% Position vector
r = a.*(1-e.^2)./(1+e.*cos(f)) .* R;

% Velocity vector
v = sqrt(mu./(a.*(1-e.^2))) .* ( e.*sin(f).*R + ( 1+e.*cos(f) ).*S );

end

== matlab function main/Real physics/Rotational dynamic/getGamma0/MATLAB Function4 ==
  data: vG0 input; Gamma0 output
function Gamma0 = getGammaZero(vG0)

m = Spacecraft.str.mass;
J = Spacecraft.str.inertia;
G_O = Spacecraft.str.com;
omega0 = Spacecraft.initialAngularSpeed;

Gamma0 = J*omega0+m*cross(G_O,vG0);

== matlab function main/Real physics/Rotational dynamic/Kinematics with quaternions/MATLAB Function1 ==
  data: omega input size=[3 1]; Omega output size=[4 4]
function Omega = getOmega(omega)
    % Considering the quaternion q = a + i x + j y + k z
    % While in class we used the following convention:
    %   q_vec = [x y z a]'
    % MATLAB use a different convention:
    %   q_vec = [a x y z]'
    % For this reason the following matrix is different from the one we seen
    
    Omega = [         0 -omega(1)  -omega(2) -omega(3) ;
                      0         0   omega(3) -omega(2) ;
                      0         0          0  omega(1) ;
                      0         0          0         0 ];
    Omega = Omega - Omega';
end

== matlab function main/Real physics/Solar radiation pressure (torque only)/MATLAB Function1 ==
  data: time input; SunDirection_NF output
function SunDirection_NF = SunPosition(time)
eps = deg2rad(23.45);
nSun = 2*pi/(365.25*24*3600);
SunDirection_NF = [cos(nSun*time) sin(nSun*time)*cos(eps) sin(nSun*time)*sin(eps)]';

== matlab function main/Real physics/Solar radiation pressure (torque only)/MATLAB Function2 ==
  data: P input; A input; r input; n input; rhod input; rhos input; Re input; sunDir_BF input; scPos_BF input; F output; T output; umbra output
function [F,T,umbra] = SRPTorque(P,A,r,n,rhod,rhos,Re,sunDir_BF,scPos_BF)
    
    F = [0 0 0]';
    T = [0 0 0]';
    
    R = norm(scPos_BF);
    scDir_BF = scPos_BF / R;
    if dot(-sunDir_BF,scDir_BF) < cos(asin(Re/R))
        umbra = false;
        for i=1:numel(A)
           appo = dot(sunDir_BF,n(:,i));
           if appo > 0
               f = -P*A(i)*appo*(...
                     (1-rhos(i))*sunDir_BF + ...
                     2*rhos(i)*appo*n(:,i) + ...
                     2/3*rhod(i)*n(:,i)...
                   );
               F = F + f;
               T = T + cross(r(:,i),f);
           end
        end
    else
        umbra = true;
    end
end

== matlab function main/Real physics/Gravity gradient/MATLAB Function ==
  data: mu input; J input; position_IF input; torque_IF output
function torque_IF = gravityGradient(mu,J,position_IF)

R = norm(position_IF);
c = position_IF / R;

torque_IF = 3*mu/R^3*[(J(3)-J(2))*c(2)*c(3) (J(1)-J(3))*c(1)*c(3) (J(2)-J(1))*c(1)*c(2)]';

== matlab function main/MPC/MATLAB Function ==
  data: u input; y output
function y = fcn(u)

y = u;

== matlab function main/Ideal control law/MATLAB Function5 ==
  data: om input; e output
function e = fcn(om)

e = sqrt(om(1)^2+om(2)^2+om(3)^2) * 180 / pi * 2;

== matlab function main/Subsystem1/Sun sensor reading1/Subsystem/MATLAB Function2 ==
  data: theta input; q output size=[1 4]; e input
function q = crossBoresightRotation(theta,e)

q = [cos(theta/2) sin(theta/2)*[e(1) e(2)] 0];

== matlab function main/Control allocator/Subsystem3/MATLAB Function ==
  data: u input; y output
function y = fcn(u)
if u > 0.5
    y = 1;
else
    y = 0;
end

== matlab function main/Control allocator/Subsystem3/MATLAB Function1 ==
  data: u input; y output
function y = fcn(u)
if u > 0.5
    y = 1;
else
    y = 0;
end

== matlab function main/Control allocator/Subsystem3/MATLAB Function2 ==
  data: u input; y output
function y = fcn(u)
if u > 0.5
    y = 1;
else
    y = 0;
end

== matlab function main/Control allocator/Subsystem3/MATLAB Function3 ==
  data: u input; y output
function y = fcn(u)
if u > 0.5
    y = 1;
else
    y = 0;
end

== matlab function main/Control allocator/MATLAB Function ==
  data: u input; y output
function y = fcn(u)
if u > 0.5
    y = 1;
else
    y = 0;
end

== matlab function main/Control allocator/MATLAB Function1 ==
  data: u input; y output
function y = fcn(u)
if u > 0.5
    y = 1;
else
    y = 0;
end

== matlab function main/Control allocator/MATLAB Function2 ==
  data: u input; y output
function y = fcn(u)
if u > 0.5
    y = 1;
else
    y = 0;
end

== matlab function main/Control allocator/MATLAB Function4 ==
  data: u input; y output
function y = fcn(u)
if u > 0.5
    y = 1;
else
    y = 0;
end

== matlab function main/Star sensor/Vector 2 angles/Subsystem/MATLAB Function ==
  data: theta input; q output
function q = aboutBoresightRotation(theta)

q = [cos(theta/2) 0 0 sin(theta/2)];

== matlab function main/Real physics/Air drag/MATLAB Function ==
  data: F output; rho input; relVel input; T output; Spacecraft input
function [F,T] = getAirTorqueAndForce(rho, relVel, Spacecraft)

F = zeros(3,1);
T = zeros(3,1);

relVelMag = norm(relVel);
relVelDir = relVel/relVelMag;

for i = 1:size(Spacecraft.surfaces_normalToSurface,2)
    N_i = Spacecraft.surfaces_normalToSurface(:,i);
    A_i = Spacecraft.surfaces_area(:,i);
    r_i = Spacecraft.surfaces_position(:,i);
    Cd_i = Spacecraft.surfaces_Cd(i);
    
    F_i = dot(relVelDir,N_i);
    if F_i > 0
       F_i = F_i * 1/2*rho*Cd_i*relVelMag^2*A_i;
    else
       F_i = 0;
    end
    
    F = F - F_i * relVelDir;
    T = T - cross(r_i + Spacecraft.geometricCenter, F_i * relVelDir);
end

== matlab function main/Star sensor/Vector 2 angles/Subsystem/MATLAB Function1 ==
  data: theta input; q output size=[1 4]; e input
function q = crossBoresightRotation(theta,e)

q = [cos(theta/2) sin(theta/2)*[e(1) e(2)] 0];

== matlab function main/Star sensor/Vector 2 angles1/Subsystem/MATLAB Function ==
  data: theta input; q output
function q = aboutBoresightRotation(theta)

q = [cos(theta/2) 0 0 sin(theta/2)];

== matlab function main/Star sensor/Vector 2 angles1/Subsystem/MATLAB Function1 ==
  data: theta input; q output size=[1 4]; e input
function q = crossBoresightRotation(theta,e)

q = [cos(theta/2) sin(theta/2)*[e(1) e(2)] 0];

== matlab function main/Star sensor/Vector 2 angles2/Subsystem/MATLAB Function ==
  data: theta input; q output
function q = aboutBoresightRotation(theta)

q = [cos(theta/2) 0 0 sin(theta/2)];

== matlab function main/Star sensor/Vector 2 angles2/Subsystem/MATLAB Function1 ==
  data: theta input; q output size=[1 4]; e input
function q = crossBoresightRotation(theta,e)

q = [cos(theta/2) sin(theta/2)*[e(1) e(2)] 0];

== matlab function main/Star sensor/Vector 2 angles3/Subsystem/MATLAB Function ==
  data: theta input; q output
function q = aboutBoresightRotation(theta)

q = [cos(theta/2) 0 0 sin(theta/2)];

== matlab function main/Star sensor/Vector 2 angles3/Subsystem/MATLAB Function1 ==
  data: theta input; q output size=[1 4]; e input
function q = crossBoresightRotation(theta,e)

q = [cos(theta/2) sin(theta/2)*[e(1) e(2)] 0];

== matlab function main/Real physics/Magnetic dipole/Subsystem2/MATLAB Function ==
  data: RAGreenwich input; Bth output; RA input; dec input; r input; Bph output; Br output
function [Bth, Bph, Br] = magneticField(RAGreenwich,RA,dec,r)

ph = RA - RAGreenwich;
th = pi/2 - dec;

Bth = (1.0./r.^5.*(sin(th.*2.0).*(cos(th.*2.0).*5.0e-1-5.0e-1).*4.99040610822406e-6+cos(th).^3.*sin(th).*1.330774962193083e-5+sin(th).*(sin(ph.*4.0).*9.8e-8-cos(ph.*3.0).*4.21e-7).*sqrt(-(cos(th).^2-1.0).^3).*2.091650066335189+sin(th.*2.0).*sqrt((cos(th.*2.0)-1.0).^2).*(cos(ph.*2.0).*2.91e-7-sin(ph.*4.0).*2.32e-7).*1.956559480312316+(sin(ph.*4.0).*2.62e-7+cos(ph).*7.820000000000001e-7).*sqrt(-cos(th).^2+1.0).*(sin(th).*1.728e+4-sin(th).^3.*2.016e+4).*8.235098073355155e-4+cos(ph.*4.0+1.202954787756519).*cos(th).*sin(th).*1.0./sqrt((cos(th).^2-1.0).^4).*(cos(th).^2-1.0).^3.*9.542005816388921e-7-cos(th).^2.*sin(th).*(sin(ph.*4.0).*9.8e-8-cos(ph.*3.0).*4.21e-7).*1.0./sqrt(-(cos(th).^2-1.0).^3).*(cos(th).^2-1.0).^2.*6.274950199005567+cos(th).*sin(th).*(sin(ph.*4.0).*2.62e-7+cos(ph).*7.820000000000001e-7).*1.0./sqrt(-cos(th).^2+1.0).*(cos(th).*2.88e+3-cos(th).^3.*6.72e+3).*8.235098073355155e-4+cos(th).*sin(th).*1.0./sqrt((cos(th).^2-1.0).^2).*(cos(th).^2.*2.016e+4-2.88e+3).*(cos(th).^2-1.0).*(cos(ph.*2.0).*2.91e-7-sin(ph.*4.0).*2.32e-7).*3.882062460937135e-4).*6.732293806813025e+22-1.0./r.^3.*(cos(th).*sin(th).*9.321081589601071e-6-(sin(ph.*2.0).*cos(th).^2.*sin(th).*1.81892728695232e+32-cos(ph).*cos(th).^2.*sin(th).*2.373252326015039e+32).*1.0./sqrt(cos(th).^2.*-3.333333333333333e+32+3.333333333333333e+32).*4.096e-22+sin(th).*(sin(ph.*2.0).*2.23509785020701e+32-cos(ph).*2.91625245820728e+32).*sqrt(cos(th.*2.0).*-1.666666666666667e+32+1.666666666666667e+32).*1.0e-54-cos(ph.*2.0+2.470721701870364e-1).*cos(th).*sin(th).*1.0./sqrt((cos(th).^2-1.0).^2).*(cos(th).^2-1.0).*3.009908636487161e-6).*1.654913786623872e+15+1.0./r.^4.*(sin(th).*1.127693894636306e-5-sin(th).^3.*1.409617368295383e-5-sin(th.*2.0).*(sin(ph.*3.0).*2.63e-7+cos(ph).*2.268e-6).*sqrt(cos(th.*2.0).*-8.333333333333333e-2+8.333333333333333e-2).*7.5+sin(th).*sqrt((cos(th).^2-1.0).^2).*(cos(ph.*2.0).*1.249e-6+sin(ph.*3.0).*3.02e-7).*1.936491673103708+sin(th.*2.0).*(sin(ph.*3.0).*2.63e-7+cos(ph).*2.268e-6).*1.0./sqrt(cos(th.*2.0).*-8.333333333333333e-2+8.333333333333333e-2).*(cos(th.*2.0).*1.8e+2+1.08e+2).*1.736111111111111e-3-cos(ph.*3.0+4.857633442146602e-1).*cos(th).*sin(th).*1.0./sqrt(-(cos(th).^2-1.0).^3).*(cos(th).^2-1.0).^2.*2.062427726006417e-6+cos(th).^2.*sin(th).*1.0./sqrt((cos(th).^2-1.0).^2).*(cos(th).^2-1.0).*(cos(ph.*2.0).*1.249e-6+sin(ph.*3.0).*3.02e-7).*3.872983346207417).*1.055526685427583e+19-1.0./r.^2.*1.0./sqrt(cos(th.*2.0).*-5.0e-1+5.0e-1).*(sin(th).*sqrt(cos(th.*2.0).*-5.0e-1+5.0e-1).*2.623542934897388e+32-cos(ph+1.246284126936341).*sin(th.*2.0).*1.753390827662575e+31).*4.151466264519241e-26)./r;
Bph = (1.0./r.^3.*(cos(ph.*2.0-1.32372415660786).*sqrt((cos(th).^2-1.0).^2).*3.009908636487161e-6+cos(th).*(cos(ph.*2.0).*4.470195700414021e+32+sin(ph).*2.91625245820728e+32).*sqrt(cos(th.*2.0).*-1.666666666666667e+32+1.666666666666667e+32).*1.0e-54).*1.654913786623872e+15+1.0./r.^4.*(cos(ph.*3.0-1.085032982580236).*sqrt(-(cos(th).^2-1.0).^3).*2.062427726006417e-6+(cos(ph.*3.0).*7.89e-7-sin(ph).*2.268e-6).*(cos(th).^2.*3.6e+2-7.2e+1).*sqrt(cos(th).^2.*-1.666666666666667e+32+1.666666666666667e+32).*6.588078458684124e-19+cos(th).*(sin(ph.*2.0).*2.498e-6-cos(ph.*3.0).*9.060000000000001e-7).*sqrt((cos(th).^2-1.0).^2).*1.936491673103708).*1.055526685427583e+19+1.0./r.^5.*(cos(ph.*4.0-3.678415390383772e-1).*sqrt((cos(th).^2-1.0).^4).*9.542005816388921e-7+(cos(ph.*4.0).*1.048e-6-sin(ph).*7.820000000000001e-7).*sqrt(-cos(th).^2+1.0).*(cos(th).*2.88e+3-cos(th).^3.*6.72e+3).*8.235098073355155e-4-cos(th).*sqrt(-(cos(th).^2-1.0).^3).*(cos(ph.*4.0).*3.92e-7+sin(ph.*3.0).*1.263e-6).*2.091650066335189+sqrt((cos(th).^2-1.0).^2).*(cos(th).^2.*2.016e+4-2.88e+3).*(cos(ph.*4.0).*9.280000000000001e-7+sin(ph.*2.0).*5.82e-7).*1.941031230468567e-4).*6.732293806813025e+22-1.0./r.^2.*cos(ph-3.24512199858556e-1).*sqrt(-cos(th).^2+1.0).*1.45582857391173e+6)./(r.*sin(th));
Br  = 1.0./r.^5.*(cos(th).*(cos(th).^2-1.0).*2.819234736590765e-6+cos(th).^3.*1.879489824393843e-6+cos(ph.*3.0+4.857633442146602e-1).*sqrt(-(cos(th).^2-1.0).^3).*6.874759086688057e-7-(sin(ph.*3.0).*2.63e-7+cos(ph).*2.268e-6).*(cos(th).^2.*3.6e+2-7.2e+1).*sqrt(cos(th).^2.*-1.666666666666667e+32+1.666666666666667e+32).*6.588078458684124e-19+cos(th).*sqrt((cos(th).^2-1.0).^2).*(cos(ph.*2.0).*1.249e-6+sin(ph.*3.0).*3.02e-7).*1.936491673103708).*4.22210674171033e+19+1.0./r.^6.*(cos(ph.*4.0+1.202954787756519).*sqrt((cos(th).^2-1.0).^4).*2.38550145409723e-7+(cos(th).^2-1.0).^2.*4.99040610822406e-7+cos(th).^4.*1.330774962193083e-6+cos(th).^2.*(cos(th).^2-1.0).*3.992324886579248e-6-(sin(ph.*4.0).*2.62e-7+cos(ph).*7.820000000000001e-7).*sqrt(-cos(th).^2+1.0).*(cos(th).*2.88e+3-cos(th).^3.*6.72e+3).*8.235098073355155e-4+cos(th).*(sin(ph.*4.0).*9.8e-8-cos(ph.*3.0).*4.21e-7).*sqrt(-(cos(th).^2-1.0).^3).*2.091650066335189+sqrt((cos(th).^2-1.0).^2).*(cos(th).^2.*2.016e+4-2.88e+3).*(cos(ph.*2.0).*2.91e-7-sin(ph.*4.0).*2.32e-7).*1.941031230468567e-4).*3.366146903406512e+23-1.0./r.^4.*(cos(th).^2.*4.660540794800535e-6-cos(ph.*2.0+2.470721701870364e-1).*sqrt((cos(th).^2-1.0).^2).*1.504954318243581e-6+cos(th).*(sin(ph.*2.0).*2.23509785020701e+32-cos(ph).*2.91625245820728e+32).*sqrt(cos(th.*2.0).*-1.666666666666667e+32+1.666666666666667e+32).*1.0e-54-1.553513598266845e-6).*4.964741359871617e+15-1.0./r.^3.*(cos(th).*2.178309997548861e+32+cos(ph+1.246284126936341).*sqrt(-cos(th).^2+1.0).*2.911657147823461e+31).*1.0e-25;

== matlab function main/Real physics/Magnetic dipole/Subsystem2/MATLAB Function1 ==
  data: RA output; dec output; r_NF input; r output
function [RA,dec,r] = car2sid(r_NF)
RA  = atan2(r_NF(2),r_NF(1));
r = norm(r_NF);
dec = asin(r_NF(3)/r);

== matlab function main/Real physics/Magnetic dipole/Subsystem2/Subsystem1/MATLAB Function2 ==
  data: RA input; q output size=[1 4]
function q = getq1(RA)
q = [cos(RA/2) 0 0 sin(RA/2)];

== matlab function main/Real physics/Magnetic dipole/Subsystem2/Subsystem1/MATLAB Function3 ==
  data: dec input; q output size=[1 4]
function q = getq2(dec)
q = [cos(pi/4 - dec/2) 0 sin(pi/4 - dec/2) 0];

== matlab function main/Subsystem1/Sun sensor reading/Subsystem/MATLAB Function ==
  data: theta input; q output
function q = aboutBoresightRotation(theta)

q = [cos(theta/2) 0 0 sin(theta/2)];

== matlab function main/Subsystem1/Sun sensor reading2/Subsystem/MATLAB Function ==
  data: theta input; q output
function q = aboutBoresightRotation(theta)

q = [cos(theta/2) 0 0 sin(theta/2)];

== matlab function main/MATLAB Function ==
  data: t input; q output; omega output
function [q,omega] = fcn(t)

om = 1/3600;
q = [cos(om*t/2) 0 sin(om*t/2) 0]';
omega = [0 1 0]'*om;

== matlab function main/Subsystem1/Sun sensor reading2/Subsystem/MATLAB Function2 ==
  data: theta input; q output size=[1 4]; e input
function q = crossBoresightRotation(theta,e)

q = [cos(theta/2) sin(theta/2)*[e(1) e(2)] 0];

== matlab function main/Subsystem1/Sun sensor reading3/Subsystem/MATLAB Function ==
  data: theta input; q output
function q = aboutBoresightRotation(theta)

q = [cos(theta/2) 0 0 sin(theta/2)];

== matlab function main/Subsystem1/Sun sensor reading3/Subsystem/MATLAB Function2 ==
  data: theta input; q output size=[1 4]; e input
function q = crossBoresightRotation(theta,e)

q = [cos(theta/2) sin(theta/2)*[e(1) e(2)] 0];
